simulink model "SimulazioneRobot"  (R2025b)
settings: Solver=ode4  StartTime=0.0  StopTime=10  FixedStep=0.001  MaxStep=0.1  RelTol=1e-3  AbsTol=1e-3  EnableMultiTasking=on
values from neighbouring files (symbols this model uses):
  dq0_pd = zeros(nDOF, 1)    [setup_simscape.m]    (also in setup_simscape_feedforward.m; setup_simulink.m)
  kd = evalin('base','kd')    [analisi_robot.m]    (also in setup_simscape.m = 6; setup_simulink.m = 0.18)
  ki = evalin('base','ki')    [analisi_robot.m]    (also in setup_simscape.m = 2; setup_simulink.m = 2.7)
  kp = evalin('base','kp')    [analisi_robot.m]    (also in setup_simscape.m = 5; setup_simulink.m = 0.9)
  q0_pd = qinit    [setup_simscape.m]    (also in setup_simscape_feedforward.m; setup_simulink.m)
libraries: instrumentseriallib x2
settings Model: ExtModeTrigDuration=2  Creator=luca-callegari  LastModifiedBy=User
settings SolverCC: AutoInsertRateTranBlk=on
settings OptimizationCC: EnhancedBackFolding=on  PassReuseOutputArgsAs=Individual arguments  ZeroExternalMemoryAtStartup=off  ZeroInternalMemoryAtStartup=off  MaxStackSize=64  OptimizeBlockOrder=speed  DifferentSizesBufferReuse=on  OptimizationCustomize=off  EfficientTunableParamExpr=on
settings DebuggingCC: ParameterTunabilityLossMsg=error
settings HardwareCC: ProdBitPerInt=16.0  ProdBitPerPointer=16.0  ProdBitPerSizeT=16.0  ProdBitPerPtrDiffT=16.0  ProdLargestAtomicFloat=None  ProdWordSize=8.0  ProdHWDeviceType=Atmel->AVR  UseEmbeddedCoderFeatures=off
settings SFSimCC: MATLABDynamicMemAlloc=off
settings RTWCC: SystemTargetFile=ert.tlc  HardwareBoard=Arduino Uno  TemplateMakefile=ert_default_tmf  Toolchain=Arduino AVR  BuildConfiguration=Faster Runs  Description=Embedded Coder
settings CodeAppCC: ForceParamTrailComments=on  IgnoreCustomStorageClasses=off  OperatorAnnotations=on  SimulinkDataObjDesc=on  SFDataObjDesc=on  InsertBlockDesc=on
settings ERTTargetCC: ExtModeTransport=3.0  ExtModeStaticAlloc=on  ExtModeAutomaticAllocSize=off  ExtModeStaticAllocSize=250.0  ExtModeMexFile=ext_xcp  ExtModeIntrfLevel=Level2 - Open  InlinedParameterPlacement=Hierarchical  SupportContinuousTime=on  SupportNonInlinedSFcns=on  SupportVariableSizeSignals=on

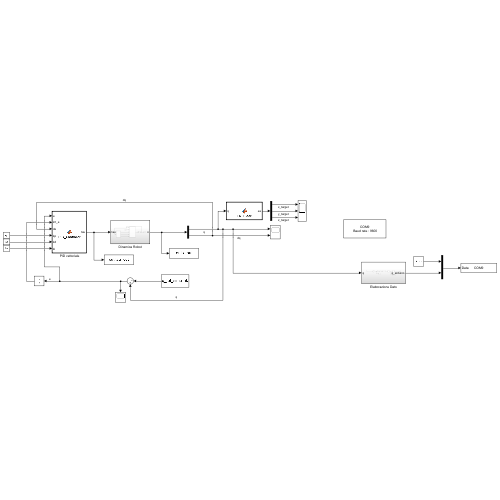
[thumbnail: Simulink's stored preview of the top-level diagram]
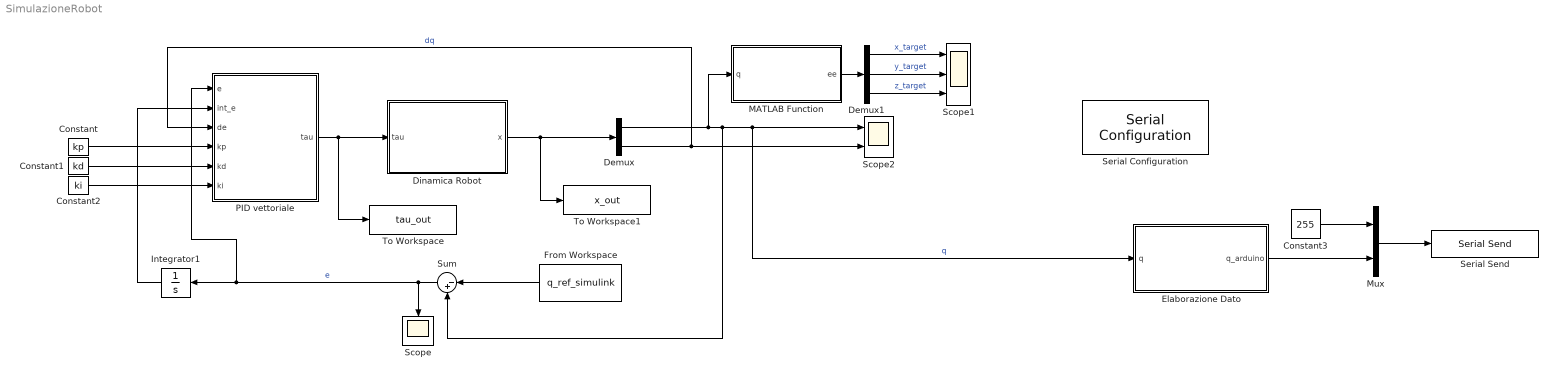
== system SimulazioneRobot ==
  " PID vettoriale" : MATLAB Function  TreatAsAtomicUnit=on
  Constant : Constant  Value=kp
  Constant1 : Constant  Value=kd
  Constant2 : Constant  Value=ki
  Constant3 : Constant  Value=255  OutDataTypeStr=uint8
  Demux : Demux  Outputs=2
  Demux1 : Demux  Outputs=3
  Dinamica Robot : Subsystem
  Elaborazione Dato : Subsystem
  From Workspace : FromWorkspace  VariableName=q_ref_simulink
  Integrator1 : Integrator  InitialCondition=zeros(3,1)
  MATLAB Function : MATLAB Function  TreatAsAtomicUnit=on
  Mux : Mux  Inputs=2
  Scope : Scope
      settings: ActiveDisplayYMinimum=-1.9458226676345514  ActiveDisplayYMaximum=0.68832822948869388
  Scope1 : Scope  NumInputPorts=3
      settings: ActiveDisplayYMinimum=-0.026374999999999992  ActiveDisplayYMaximum=0.237375
  Scope2 : Scope  NumInputPorts=2
      settings: ActiveDisplayYMinimum=-0.97787229242596907  ActiveDisplayYMaximum=2.45011994104577  DataLoggingVariableName=ScopeData2
  Serial Configuration : instrumentseriallib/Serial Configuration  Priority=-200000  PortSel=COM9  Port=COM9  ComPort=COM9  BaudRate=9600  DataBits=8  Parity=none  StopBits=1  ByteOrder=little-endian  FlowControl=none  Timeout=10  SimulateUsing=Interpreted execution  BlockInModel=on  aMode=1
      settings: LibrarySourceBlock=c2000lib/Host Communication/Serial Configuration
  Serial Send : instrumentseriallib/Serial Send  Priority=1  PortSel=COM9  Port=COM9  ComPort=COM9  Header=[]  Terminator=<none>  CustomTerminator=[]  EnableBlockingMode=on  SimulateUsing=Interpreted execution  BlockInModel=on  aMode=1
      settings: LibrarySourceBlock=c2000lib/Host Communication/Serial Send
  Sum : Sum  Inputs=|-+
  To Workspace : ToWorkspace  VariableName=tau_out  SaveFormat=Structure With Time  SampleTime=-1
  To Workspace1 : ToWorkspace  VariableName=x_out  SaveFormat=Structure With Time  SampleTime=-1
  wires:
  From Workspace/1 -> Sum/1
  Demux/1 -> Sum/2, Elaborazione Dato/1(q), Scope2/1, MATLAB Function/1(q)  "q"
  Constant/1 -> " PID vettoriale"/4(kp)
  Constant1/1 -> " PID vettoriale"/5(kd)
  Constant2/1 -> " PID vettoriale"/6(ki)
  Demux/2 -> Scope2/2, " PID vettoriale"/3(de)  "dq"
  Sum/1 -> Scope/1, " PID vettoriale"/1(e), Integrator1/1  "e"
  MATLAB Function/1(ee) -> Demux1/1
  Integrator1/1 -> " PID vettoriale"/2(int_e)
  " PID vettoriale"/1(tau) -> To Workspace/1, Dinamica Robot/1(tau)
  Dinamica Robot/1(x) -> To Workspace1/1, Demux/1
  Demux1/1 -> Scope1/1  "x_target"
  Demux1/2 -> Scope1/2  "y_target"
  Demux1/3 -> Scope1/3  "z_target"
  Constant3/1 -> Mux/1
  Elaborazione Dato/1(q_arduino) -> Mux/2
  Mux/1 -> Serial Send/1

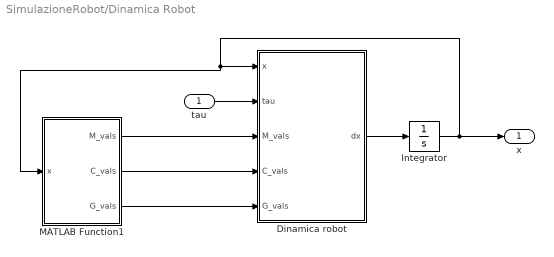
== system SimulazioneRobot/Dinamica Robot ==
  tau : Inport
  " Dinamica robot" : MATLAB Function  TreatAsAtomicUnit=on
  Integrator : Integrator  InitialCondition=[q0_pd; dq0_pd]
  MATLAB Function1 : MATLAB Function  TreatAsAtomicUnit=on
  x : Outport
  wires:
  " Dinamica robot"/1(dx) -> Integrator/1
  tau/1 -> " Dinamica robot"/2(tau)
  MATLAB Function1/2(C_vals) -> " Dinamica robot"/4(C_vals)
  MATLAB Function1/1(M_vals) -> " Dinamica robot"/3(M_vals)
  MATLAB Function1/3(G_vals) -> " Dinamica robot"/5(G_vals)
  Integrator/1 -> x/1, MATLAB Function1/1(x), " Dinamica robot"/1(x)

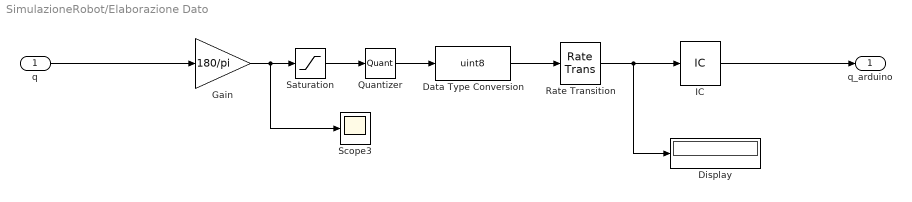
== system SimulazioneRobot/Elaborazione Dato ==
  q : Inport
  Data Type Conversion : DataTypeConversion  OutDataTypeStr=uint8  SaturateOnIntegerOverflow=off  RndMeth=Floor
  Display : Display
  Gain : Gain  Gain=180/pi
  IC : InitialCondition  Value=0
  Quantizer : Quantizer  QuantizationInterval=1
  Rate Transition : RateTransition  OutPortSampleTime=0.001
  Saturation : Saturate  UpperLimit=180  LowerLimit=0  OutDataTypeStr=single
  Scope3 : Scope
      settings: ActiveDisplayYMinimum=-1  ActiveDisplayYMaximum=1  DataLoggingVariableName=ScopeData3
  q_arduino : Outport
  wires:
  Gain/1 -> Scope3/1, Saturation/1
  q/1 -> Gain/1
  Data Type Conversion/1 -> Rate Transition/1
  Saturation/1 -> Quantizer/1
  Quantizer/1 -> Data Type Conversion/1
  Rate Transition/1 -> IC/1, Display/1
  IC/1 -> q_arduino/1

== matlab function SimulazioneRobot/Dinamica Robot/ Dinamica robot ==
  data: x input; tau input; dx output size=[6,1]; M_vals input; C_vals input; G_vals input
% =========================================================================
%  ROBOT_DYNAMICS_BLOCK  -  Dinamica robot per blocco MATLAB Function
%  =========================================================================
%  Da incollare nel blocco "MATLAB Function" di Simulink che implementa
%  la dinamica del robot.
%
%  Equazione del moto:
%    M(q)*ddq + C(q,dq) + G(q) = tau
%    => ddq = M(q)^{-1} * (tau - C(q,dq) - G(q))
%
%  INPUT (porte Simulink):
%    x    : stato [q1,...,qN, dq1,...,dqN]  [2*nDOF x 1]
%    tau  : coppia di controllo             [nDOF x 1]
%
%  OUTPUT (porte Simulink):
%    dx   : derivata stato [dq; ddq]        [2*nDOF x 1]
%
%  NOTA: M_func, C_func, G_func, nDOF vengono letti dal workspace
%        Simulink (definiti in setup_simulink.m).
% =========================================================================

function dx = Dinamica_robot(x, tau, M_vals, C_vals, G_vals)

    % Le matrici M, C, G vengono pre-calcolate fuori e passate come input
    % Il blocco che le calcola e' "Calcola MCG"

    % Dimensione della variabile q(t)
    nDOF = 3;

    % Notare che q non serve perché serviva solo per valutare M_vals, 
    % C_vals, G_vals... cosa fatta nella matlab function "Calcola MCG"
    q = x(1:nDOF);
    dq = x(nDOF+1:2*nDOF);

    % Dichiarazione esplicita per Simulink
    ddq = zeros(nDOF, 1);
    dx  = zeros(2*nDOF, 1);

    % Smorzamento numerico: stabilizza il solver senza alterare la fisica
    % epsilon piccolo non cambia il comportamento reale del sistema
    epsilon = 1e-6;
    M_reg   = M_vals + epsilon * eye(nDOF);

    % Formula inversa per determinare la ddq della formula generale (usando
    % l'ingresso con PID)
    ddq = M_reg\(tau-C_vals-G_vals);

    dx = [dq; ddq];

end

== matlab function SimulazioneRobot/ PID vettoriale ==
  data: e input; int_e input; tau output; de input; kp input; kd input; ki input
%     - Porte input:  e [3x1], int_e [3x1], de [3x1], kp, kd, ki (scalari)
%     - Porta output: tau [3x1]
%     - kp, kd, ki vengono da blocchi Constant con Value = 'kp', 'kd', 'ki'

function tau = PID_Controller(e, int_e, de, kp, kd, ki)

    tau = -kp*e - kd*de - ki*int_e;

end

== matlab function SimulazioneRobot/MATLAB Function ==
  data: q input; ee output size=[3;1]
%     - Porta input:  q [3x1]
%     - Porta output: ee [3x1] = [x,y,z]

function ee = FK_Block(q)
% Chiama direttamente il file generato 
    ee = robot_f_generated(q(1), q(2), q(3));
end

== matlab function SimulazioneRobot/Dinamica Robot/MATLAB Function1 ==
  data: x input; M_vals output size=[3,3]; C_vals output size=[3,1]; G_vals output size=[3,1]
function [M_vals, C_vals, G_vals] = Calcola_MCG(x)
    % Chiama direttamente i file generati 
    M_vals = robot_M_generated(x);
    C_vals = robot_C_generated(x);
    G_vals = robot_G_generated(x);
end
